simulink model "Coulombs"  (R2024a)
settings: Solver=VariableStepAuto  StartTime=0.0  StopTime=100.0  RelTol=1e-3
undefined symbols (not defined in the file or in its folder): Ion, Lithium
libraries: simulink x1, spsBatteryLib x1, spsControlledCurrentSourceLib x1, spsCurrentMeasurementLib x1, spsVariableCapacitorLib x1, spsVoltageMeasurementLib x1, sps_lib x1
settings Model: Creator=DELL  LastModifiedBy=DELL

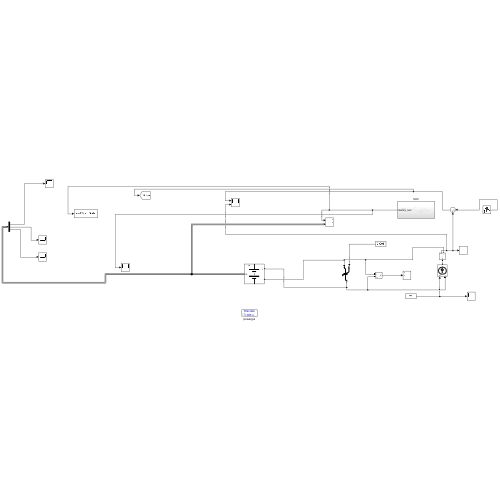
[thumbnail: Simulink's stored preview of the top-level diagram]
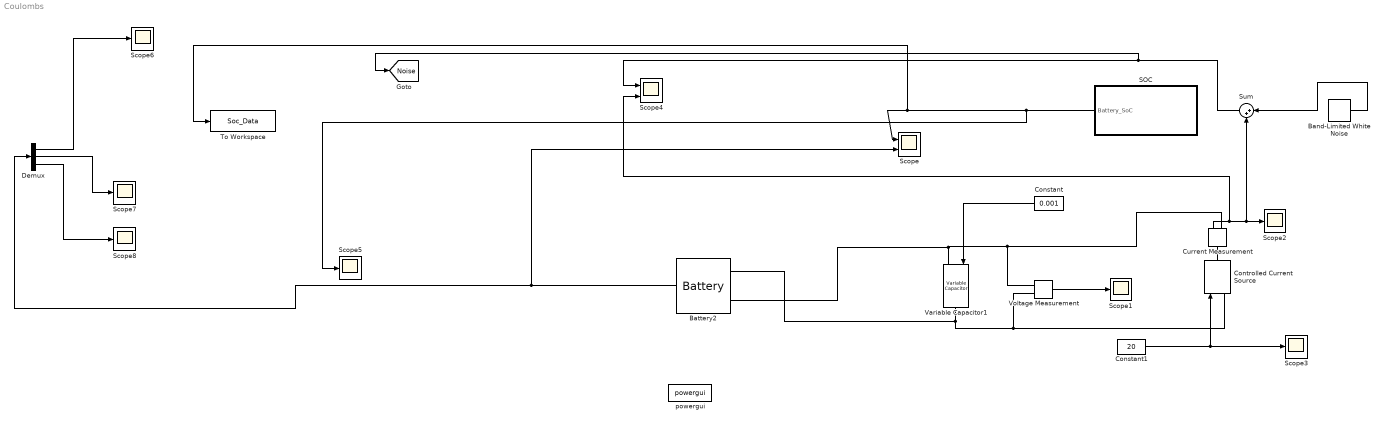
== system Coulombs ==
  Band-Limited White Noise : simulink/Sources/Band-Limited White Noise  Cov=100  Ts=1  seed=12345
  Battery2 : spsBatteryLib/Battery  BatType=Lithium-Ion  ShowTempParam=off  ThermalPreset=no  ShowAgeParam=off  NomV=3.6  NomQ=4.5  SOC=70  Batt_Tr=30  PresetModel=on  MaxQ=4.5  MinV=2.7  FullV=4.1904  Dis_rate=1.9565  R=0.008  Normal_OP=4.0696  expZone="[3.8894     0.22109]"  current=[6.5 13 32.5]  Units=Time  Tci=20  NomT=20  T2=-30  MaxQ2=4.8  FullV2=7.1  Normal_OP2=5.655  expZone2="[6.58           1]"  Rca=0.6  ti=2000  Dp=0  Neq0=0  Tsim=1e6  Ta1=25  Qeol=5.4*0.9  Reol=0.013333*1.2  Char_age=[2.3478, 3]  Dis_age=[2.3478, 10]  N1=1500  N2=10500  N3=1000  N4=1400  Ta2=45  N5=950
  Constant : Constant  Value=0.001
  Constant1 : Constant  Value=20
  Controlled Current Source : spsControlledCurrentSourceLib/Controlled Current Source  Initialize=on  Source_Type=AC  Amplitude=0  Phase=0  Frequency=0  Measurements=None
  Current Measurement : spsCurrentMeasurementLib/Current Measurement  PhasorSimulation=off  OutputType=Complex  PSBequivalent=0
  Demux : Demux  Outputs=3
  SOC : Subsystem
  Scope : Scope  NumInputPorts=2
  Scope{1..3,5..8} (7 alike) : Scope
  Scope4 : Scope  NumInputPorts=2
  Sum : Sum  Inputs=|++
  To Workspace : ToWorkspace  VariableName=Soc_Data  SaveFormat=Timeseries  SampleTime=-1
  Variable Capacitor1 : spsVariableCapacitorLib/Variable Capacitor  methode=Backward Euler  Cabsmin=1e-9  Initialize=on  vC0=0.001  C0=1e-6  iC0=-0.125
      settings: LibrarySourceBlock=sps_lib/Passives/Variable Capacitor
  Voltage Measurement : spsVoltageMeasurementLib/Voltage Measurement  PhasorSimulation=off  OutputType=Complex  PSBequivalent=0
  powergui : sps_lib/powergui  SimulationMode=Discrete  SampleTime=0.005  frequency=60  Iterations=50  frequencyindice=0  Pbase=100e6  ErrMax=1e-4  UnitsV=kV  UnitsW=MW  buscounter=0  FunctionMessages=off  echomessages=off  EnableUseOfTLC=off  CurrentSourceSwitches=off  DisableSnubberDevices=off  DisableRonSwitches=off  DisableVfSwitches=off  DisplayEquations=off  AutomaticDiscreteSolvers=off  SolverType=Tustin  Interpol=off  ExternalGateDelay=off  methode=off  Ts=0  x0status=blocks  SPID=off  SwTol=0  HookPort=off  NonlinearTolerance=1e-4  nMaxIteration=100  ContinueOnMaxIteration=off  RestoreLinks=warning  ResistiveCurrentMeasurement=off  Frange=[0:2:500]  Ylog=off  Xlog=on  ShowGrid=off  save=off  variable=ZData  structure=0  ZoomFFT=on  StartTime=0.0  cycles=1  DisplayStyle=1  fundamental=60  FreqAxis=off  MaxFrequency=1000  frequencyindicesteady=1  RmsSteady=1  display=off
  tag scope: Noise=global
  wires:
  Constant1/1 -> Scope3/1, Controlled Current Source/1
  Band-Limited White Noise/1 -> Sum/1
  Voltage Measurement/1 -> Scope1/1
  SOC/1(Battery_SoC) -> Scope5/1, To Workspace/1, Scope/1
  Current Measurement/1 -> Scope4/2, Scope2/1, Sum/2
  Sum/1 -> [Noise], Scope4/1
  Constant/1 -> Variable Capacitor1/1
  Battery2/1 -> Scope/2, Demux/1
  Demux/1 -> Scope6/1
  Demux/2 -> Scope7/1
  Demux/3 -> Scope8/1
  connections:
  Variable Capacitor1/LConn1 -- Battery2/LConn2 -- Voltage Measurement/LConn2 -- Current Measurement/RConn1
  Controlled Current Source/LConn1 -- Battery2/LConn1 -- Variable Capacitor1/RConn1 -- Voltage Measurement/LConn1
  Current Measurement/LConn1 -- Controlled Current Source/RConn1

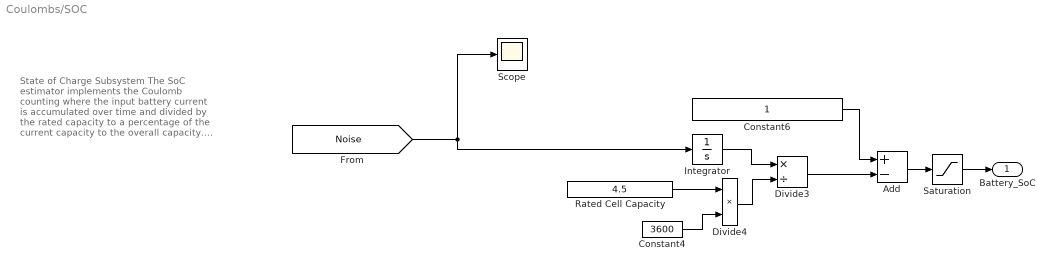
== system Coulombs/SOC ==
  note: State of Charge Subsystem
      |
      | The SoC estimator implements the Coulomb counting where the input battery current is accumulated over time and divided by the rated capacity to a percentage of the current capacity to the overall capacity. The output of this subsystem outputs the state of charge as a percentage.
  Add : Sum  Inputs=+-
  Constant4 : Constant  Value=3600
  Constant6 : Constant
  Divide3 : Product  Inputs=*/
  Divide4 : Product  Inputs=**
  Integrator : Integrator
  Rated Cell Capacity : Constant  Value=4.5  OutMin=3.2  OutMax=4.5
  Saturation : Saturate  UpperLimit=1  LowerLimit=0
  Scope : Scope
  Battery_SoC : Outport
  wires:
  Constant6/1 -> Add/1
  Divide3/1 -> Add/2
  Divide4/1 -> Divide3/2
  Rated Cell Capacity/1 -> Divide4/1
  Integrator/1 -> Divide3/1
  Constant4/1 -> Divide4/2
  [Noise] -> Integrator/1, Scope/1
  Saturation/1 -> Battery_SoC/1
  Add/1 -> Saturation/1
